simulink model "PV_Array_with_Boost"  (R2020a)
settings: Solver=ode3  StartTime=0.0  StopTime=10  FixedStep=5e-6  RelTol=1e-3
libraries: powerlib x21, powerlib_meascontrol x2, re_lib x1, eePwmGenerator x1
settings Model: Creator=Niaz  LastModifiedBy=alekh
settings DataIOCC: LimitDataPoints=on  SaveFormat=Array  ReturnWorkspaceOutputs=off
settings OptimizationCC: LifeSpan=inf
settings DebuggingCC: SFUnexpectedBacktrackingDiag=warning  SFNoUnconditionalDefaultTransitionDiag=warning  SFExecutionAtInitializationDiag=none  ArithmeticOperatorsInVariantConditions=warning
settings HardwareCC: ProdBitPerPointer=32  ProdBitPerSizeT=32  ProdBitPerPtrDiffT=32  ProdLargestAtomicFloat=None  ProdIntDivRoundTo=Undefined  ProdEndianess=Unspecified  ProdWordSize=32  ProdHWDeviceType=32-bit Generic
settings ModelReferenceCC: PropagateSignalLabelsOutOfModel=off
settings SFSimCC: SimUseLocalCustomCode=off  CustomCodeUndefinedFunction=UseInterfaceOnly
settings RTWCC: RTWUseLocalCustomCode=off
settings CodeAppCC: StateflowObjectComments=on
settings GRTTargetCC: TargetLangStandard=C89/C90 (ANSI)
settings ConfigComp: CovMetricSettings=dw  CovHtmlReporting=on  CovSaveCumulativeToWorkspaceVar=on  CovSaveSingleToWorkspaceVar=on  CovExternalEMLEnable=off
settings SimscapeCC: SimscapeNormalizeSystem=off

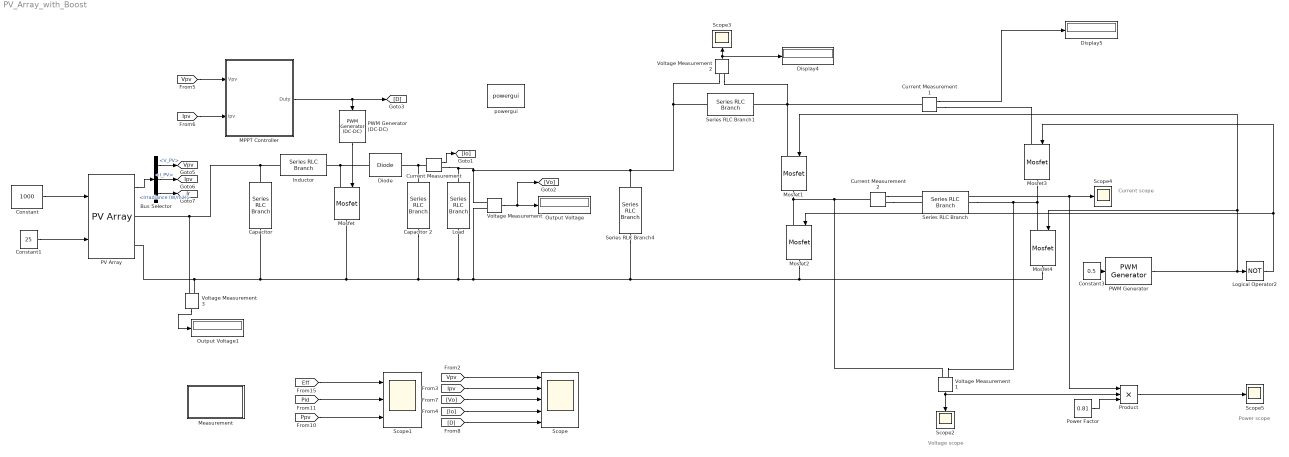
== system PV_Array_with_Boost ==
  note: Power scope
  note: Voltage scope
  note: Current scope
  Bus Selector : BusSelector  OutputSignals=V_PV,I_PV,Irradiance (W/m2)
  Capacitor : powerlib/Elements/Series RLC Branch  LConnTagsString=__new0  RConnTagsString=__new0  BranchType=C  Resistance=1e-4  Inductance=2e-3  SetiL0=off  InitialCurrent=5  Capacitance=100e-6  Setx0=off  InitialVoltage=0  Measurements=None
  Capacitor 2 : powerlib/Elements/Series RLC Branch  LConnTagsString=__new0  RConnTagsString=__new0  BranchType=C  Resistance=1e-4  Inductance=2e-3  SetiL0=off  InitialCurrent=5  Capacitance=7600*10^(-6)  Setx0=off  InitialVoltage=0  Measurements=None
  Constant : Constant  Value=1000
  Constant1 : Constant  Value=25
  Constant3 : Constant  Value=0.5
  Current Measurement : powerlib/Measurements/Current Measurement  PhasorSimulation=off  OutputType=Complex  PSBequivalent=0
  Current Measurement1 : powerlib/Measurements/Current Measurement  PhasorSimulation=off  OutputType=Complex  PSBequivalent=0
  Current Measurement2 : powerlib/Measurements/Current Measurement  PhasorSimulation=off  OutputType=Complex  PSBequivalent=0
  Diode : powerlib/Power Electronics/Diode  Ron=0.001  Lon=0  Vf=0.8  IC=0  UseSnubber=off  Rs=500  Cs=250e-9  Measurements=off
  Display4 : Display
  Display5 : Display
  Inductor : powerlib/Elements/Series RLC Branch  LConnTagsString=__new0  RConnTagsString=__new0  BranchType=L  Resistance=0.1  Inductance=1.33*10^(-3)  SetiL0=off  InitialCurrent=5  Capacitance=1e-6  Setx0=off  InitialVoltage=0  Measurements=None
  Load : powerlib/Elements/Series RLC Branch  LConnTagsString=__new0  RConnTagsString=__new0  BranchType=R  Resistance=320  Inductance=5e-5  SetiL0=off  InitialCurrent=5  Capacitance=1e-6  Setx0=off  InitialVoltage=0  Measurements=None
  Logical Operator2 : Logic  Operator=NOT  AllPortsSameDT=off  OutDataTypeStr=boolean
  MPPT Controller : MATLAB Function  TreatAsAtomicUnit=on
  Measurement : Subsystem
  Mosfet{,1..4} (5 alike) : powerlib/Power Electronics/Mosfet  Ron=0.1  Lon=0  Rd=0.01  Vfd=0  IC=0  Rs=1e5  Cs=inf  Measurements=off
  Output Voltage : Display
  Output Voltage1 : Display
  PV Array : re_lib/Solar/PV Array  Npar=1.36  Nser=20  PlotType=array @ 1000 W/m2 & specified temperatures  S_vec="[ 1000  500  100 ]"  Temp_C_vec="[ 45 25  ]"  ModuleName=User-defined  PlotWhenSelected=off  Pm=85  Ncell=60  Voc=22  Isc=5.5  Vm=17  Im=5  beta_Voc_pc=-0.36099  alpha_Isc_pc=0.102  beta_Voc=-0.079418  alpha_Isc=0.00561  IL=5.5308  I0=2.0175e-10  nI=0.59498  Rsh=85.0363  Rs=0.47595  RobustModel=off  RobustCellTemperature=25  BAL=on  Tc=1e-6  Tfilter=5e-5
  PWM Generator : eePwmGenerator/PWM Generator  CarrCount=Up  Tper=0.02  Ts=5e-5
  PWM Generator (DC-DC) : powerlib_meascontrol/Pulse & Signal Generators/PWM Generator (DC-DC)  Fsw=5000  Ts=5e-6
  Power Factor : Constant  Value=0.81
  Product : Product  Inputs=3
  Scope : Scope  NumInputPorts=5
  Scope1 : Scope  NumInputPorts=3
  Scope{2..5} (4 alike) : Scope
  Series RLC Branch : powerlib/Elements/Series RLC Branch  LConnTagsString=__new0  RConnTagsString=__new0  BranchType=RLC  Resistance=73  Inductance=1.5*10^(-6)  SetiL0=off  InitialCurrent=0  Capacitance=760*10^(-6)  Setx0=off  InitialVoltage=0  Measurements=None
  Series RLC Branch1 : powerlib/Elements/Series RLC Branch  LConnTagsString=__new0  RConnTagsString=__new0  BranchType=R  Resistance=18  Inductance=9100*10^(-6)  SetiL0=off  InitialCurrent=0  Capacitance=1e-6  Setx0=off  InitialVoltage=0  Measurements=None
  Series RLC Branch4 : powerlib/Elements/Series RLC Branch  LConnTagsString=__new0  RConnTagsString=__new0  BranchType=C  Resistance=1  Inductance=1e-3  SetiL0=off  InitialCurrent=0  Capacitance=1.19*10^(-4)  Setx0=off  InitialVoltage=0  Measurements=None
  Voltage Measurement{,1..3} (4 alike) : powerlib/Measurements/Voltage Measurement  PhasorSimulation=off  OutputType=Complex  PSBequivalent=0
  powergui : powerlib/powergui  Priority=1  SimulationMode=Discrete  SampleTime=5e-6  frequency=60  Iterations=50  frequencyindice=0  Pbase=100e6  ErrMax=1e-4  UnitsV=kV  UnitsW=MW  buscounter=0  FunctionMessages=off  echomessages=off  EnableUseOfTLC=off  CurrentSourceSwitches=off  DisableSnubberDevices=off  DisableRonSwitches=off  DisableVfSwitches=off  DisplayEquations=off  AutomaticDiscreteSolvers=off  SolverType=Tustin/Backward Euler (TBE)  Interpol=off  ExternalGateDelay=off  methode=off  Ts=100  x0status=blocks  SPID=off  SwTol=0  HookPort=off  NonlinearTolerance=1e-4  nMaxIteration=100  ContinueOnMaxIteration=off  RestoreLinks=warning  ResistiveCurrentMeasurement=off  Frange=[0:2:500]  Ylog=off  Xlog=on  ShowGrid=off  save=off  variable=ZData  structure=0  ZoomFFT=off  StartTime=0.0  cycles=1  DisplayStyle=1  fundamental=60  FreqAxis=off  MaxFrequency=1000  frequencyindicesteady=1  RmsSteady=1  display=off
  tag scope: Ipv=global, Ir=global, Vpv=global
  wires:
  PV Array/1 -> Bus Selector/1
  Voltage Measurement/1 -> [Vo], Output Voltage/1
  [Vpv] -> Scope/1
  [Ipv] -> Scope/2
  PWM Generator (DC-DC)/1 -> Mosfet/1
  [D] -> Scope/5
  [Vo] -> Scope/3
  [Io] -> Scope/4
  Current Measurement/1 -> [Io]
  Bus Selector/1 -> [Vpv]  "<V_PV>"
  Bus Selector/2 -> [Ipv]  "<I_PV>"
  Bus Selector/3 -> [Ir]  "<Irradiance (W/m2)>"
  [Pid] -> Scope1/2
  [Eff] -> Scope1/1
  [Ppv] -> Scope1/3
  [Vpv] -> MPPT Controller/1(Vpv)
  [Ipv] -> MPPT Controller/2(Ipv)
  MPPT Controller/1(Duty) -> [D], PWM Generator (DC-DC)/1
  Constant/1 -> PV Array/1
  Constant1/1 -> PV Array/2
  Power Factor/1 -> Product/3
  Current Measurement2/1 -> Scope4/1, Product/1
  PWM Generator/1 -> Logical Operator2/1, Mosfet4/1, Mosfet1/1
  Product/1 -> Scope5/1
  Current Measurement1/1 -> Display5/1
  Logical Operator2/1 -> Mosfet3/1, Mosfet2/1
  Constant3/1 -> PWM Generator/1
  Voltage Measurement1/1 -> Scope2/1, Product/2
  Voltage Measurement2/1 -> Display4/1, Scope3/1
  Voltage Measurement3/1 -> Output Voltage1/1
  connections:
  Inductor/LConn1 -- Capacitor/LConn1 -- Voltage Measurement3/LConn1 -- PV Array/RConn1
  Voltage Measurement/LConn2 -- Mosfet4/RConn1 -- Mosfet2/RConn1 -- Series RLC Branch4/RConn1 -- Load/RConn1 -- Capacitor 2/RConn1 -- Mosfet/RConn1 -- Capacitor/RConn1 -- PV Array/RConn2 -- Voltage Measurement3/LConn2
  Current Measurement/LConn1 -- Capacitor 2/LConn1 -- Diode/RConn1
  Mosfet/LConn1 -- Inductor/RConn1 -- Diode/LConn1
  Mosfet3/RConn1 -- Voltage Measurement1/LConn2 -- Series RLC Branch/RConn1 -- Mosfet4/LConn1
  Mosfet1/RConn1 -- Voltage Measurement1/LConn1 -- Current Measurement2/LConn1 -- Mosfet2/LConn1
  Current Measurement1/RConn1 -- Mosfet3/LConn1
  Current Measurement2/RConn1 -- Series RLC Branch/LConn1
  Current Measurement1/LConn1 -- Voltage Measurement2/LConn2 -- Series RLC Branch1/RConn1 -- Mosfet1/LConn1
  Current Measurement/RConn1 -- Load/LConn1 -- Series RLC Branch4/LConn1 -- Voltage Measurement2/LConn1 -- Series RLC Branch1/LConn1 -- Voltage Measurement/LConn1

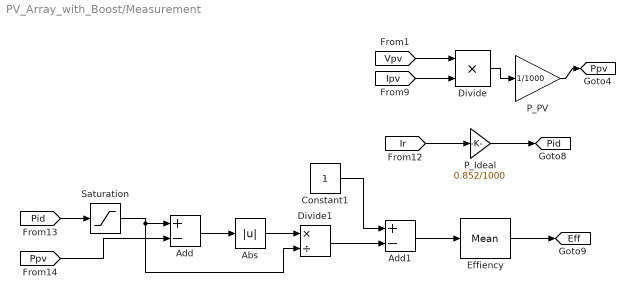
== system PV_Array_with_Boost/Measurement ==
  Abs : Abs
  Add : Sum  Inputs=+-
  Add1 : Sum  Inputs=+-
  Constant1 : Constant
  Divide : Product  Inputs=**
  Divide1 : Product  Inputs=*/
  Effiency : powerlib_meascontrol/Measurements/Mean  Freq=50  Vinit=0  Ts=50e-6
  P_Ideal : Gain  Gain=0.852/1000
  P_PV : Gain  Gain=1/1000
  Saturation : Saturate  UpperLimit=1000  LowerLimit=0.001
  tag scope: Eff=global, Pid=global, Ppv=global
  wires:
  [Ipv] -> Divide/2
  [Vpv] -> Divide/1
  [Pid] -> Saturation/1
  Add/1 -> Abs/1
  P_PV/1 -> [Ppv]
  Divide1/1 -> Add1/2
  Effiency/1 -> [Eff]
  [Ir] -> P_Ideal/1
  P_Ideal/1 -> [Pid]
  Divide/1 -> P_PV/1
  Saturation/1 -> Divide1/2, Add/1
  Add1/1 -> Effiency/1
  [Ppv] -> Add/2
  Abs/1 -> Divide1/1
  Constant1/1 -> Add1/1

== matlab function PV_Array_with_Boost/MPPT Controller ==
  data: Vpv input; Duty output; Ipv input
function Duty = PNO(Vpv, Ipv)

Delta = 125e-6;
duty_init = 0.01;
duty_min=0;
duty_max=0.99;

persistent Vold Pold duty_old;

if isempty(Vold)
    Vold=0;
    Pold=0;
    duty_old=duty_init;
end

P= Vpv*Ipv; 
dV= Vpv - Vold; 
dP= P - Pold;

if dP ~= 0
    if dP > 0
        if dV > 0
            Duty = duty_old - Delta;
        else
            Duty = duty_old + Delta;
        end
        
    else
        if dV > 0
            Duty = duty_old + Delta;
        else
            Duty = duty_old - Delta;
        end
    end
else
    Duty = duty_old;
end

if Duty >= duty_max || Duty <= duty_min
    Duty = duty_old;
end

duty_old=Duty;
Vold=Vpv;
Pold=P;
